simulink model "chldos_m"  (Simulink 7.9)
settings: Solver=ode45  SolverMode=SingleTasking  StartTime=0.0  StopTime=999999  MaxStep=10  RelTol=1e-3  AbsTol=1e-3
values from neighbouring files (symbols this model uses):
  U = st_Varia('LongNames')    [chldos_i.m]
  x0 = []    [chldos_i.m]    (also in chldos_s.m = x0)
undefined symbols (not defined in the file or in its folder): B
settings Model: Creator=M.Sparnaaij  LastModifiedBy=M.Sparnaaij
settings DataIOCC: LimitDataPoints=off  SaveOutput=off  SaveTime=off  SignalLoggingName=sigsOut
settings OptimizationCC: BooleanDataType=off
settings DebuggingCC: SaveWithParameterizedLinksMsg=none  SignalResolutionControl=TryResolveAllWithWarning  SolverPrmCheckMsg=none  MultiTaskDSMMsg=warning  MultiTaskCondExecSysMsg=none  FcnCallInpInsideContextMsg=Use local settings  StrictBusMsg=None
settings HardwareCC: TargetUnknown=on
settings RTWCC: IncludeERTFirstTime=on
settings GRTTargetCC: CombineOutputUpdateFcns=off  GRTInterface=on

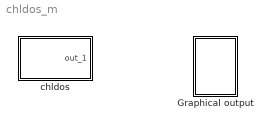
== system chldos_m ==
  Graphical output : Subsystem
      settings: OpenFcn=chldos_g
      mask Display:
      | plot(0,0,100,100,[80,20,20],[20,20,80],[80,69,60,52,45,39,33,28,24,20],[65,65,64,61,57,52,45,37,30,20])
      | disp('');
      | text(100,100,'chldos', 'horizontalAlignment', 'right', 'verticalAlignment', 'top');
  chldos : Subsystem  Description=chldos
      mask init:
      | filenaam='.\StimelaData\chldos_p.mat';
      | 
      | [Pn,Fn,Fext]=Fileprop(filenaam);
      | 
      | errstr = st_UniqName(filenaam,'filenaam=''','SubSystem','OpenFcn');
      | if errstr, error([errstr 'The filename "' filenaam '" is already in use. Choose a different filename.']), end
      | 
      | P = chldos_p(filenaam);
      | [B,x0,U]=chldos_i(filenaam);
      settings: OpenFcn=|
      | filenaam='.\StimelaData\chldos_p.mat';
      | st_ParameterInput('init',gcb,filenaam,'chldos');
      mask Display:
      | plot(0,0,100,100,[80 100],[ 50 50],[80 100],[ 55 55],[20 80 80 20 20],[10 10 90  90 10]);
      | disp('')
      | text(50,50,'chldos', 'horizontalAlignment', 'center', 'verticalAlignment', 'middle');
      | text(50,0,Fn, 'horizontalAlignment', 'center', 'verticalAlignment', 'base');

== system chldos_m/Graphical output ==
  note: plotten

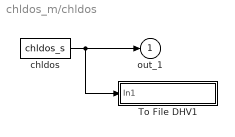
== system chldos_m/chldos ==
  To File DHV1 : Subsystem  mask(To File DHV){naam=[filenaam(1:length(filenaam)-4) '_out.sti']}
      mask prompts: naam "Naam van bestand"
      mask init:
      | set_param([gcb '/To File'],'Filename',naam);
      mask Display: disp(naam)
  chldos : S-Function  FunctionName=chldos_s  Parameters=B,x0,U,P  EnableBusSupport=off
  out_1 : Outport  InitialOutput=0
  wires:
  chldos/1 -> out_1/1, To File DHV1/1(In1)

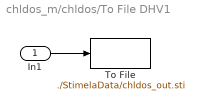
== system chldos_m/chldos/To File DHV1 ==
  In1 : Inport
  To File : ToFile  Filename=./StimelaData/chldos_out.sti  MatrixName=chldosout
  wires:
  In1/1 -> To File/1
